simulink library "uplink_4c1r_carrier_seperation_4c"  (Simulink 8.7)
settings: Solver=ode45  StartTime=0.0  StopTime=10.0  RelTol=1e-3
undefined symbols (not defined in the file or in its folder): AdvDSPBChannelOutDisplay, dspba_ChannelInVis, dspba_ChannelOutVis, dspba_internal_get_channel_ports, dspba_internal_get_demux_ports, latency, value
libraries: DSPBAPrim x11, IQ_Square x4
settings Model: Creator=bigcat  LastModifiedBy=5g

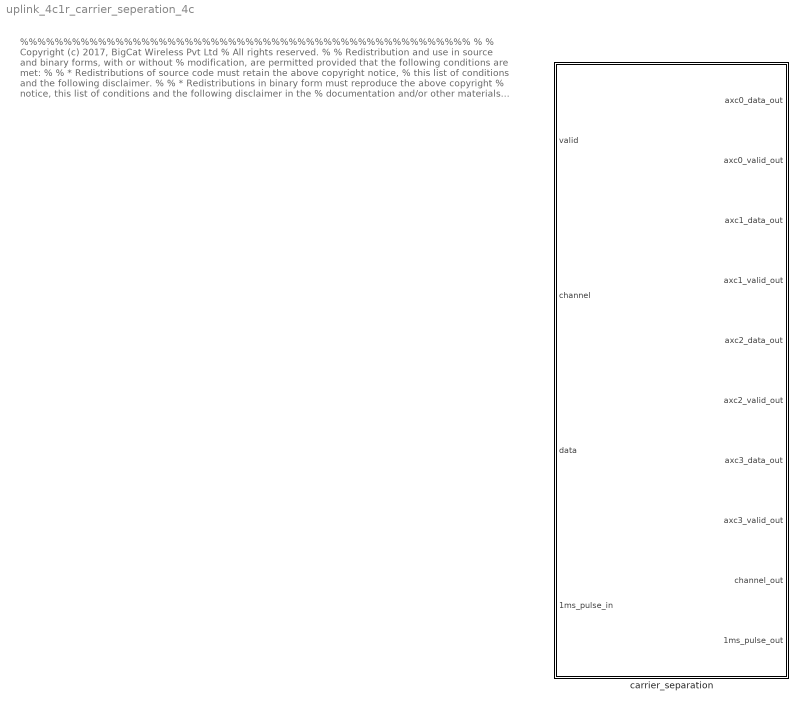
== system uplink_4c1r_carrier_seperation_4c ==
  note: %%%%%%%%%%%%%%%%%%%%%%%%%%%%%%%%%%%%%%%%%%%%%%%%%%%%
      |  %
      |  % Copyright (c) 2017, BigCat Wireless Pvt Ltd
      |  % All rights reserved.
      |  %
      |  % Redistribution and use in source and binary forms, with or without
      |  % modification, are permitted provided that the following conditions are met:
      |  %
      |  %     * Redistributions of source code must retain the above copyright notice,
      |  %       this list of conditions and the following disclaimer.
      |  %
      |  %     * Redistributions in binary form must reproduce the above copyright
      |  %       notice, this list of conditions and the following disclaimer in the
      |  %       documentation and/or other materials provided with the distribution.
      |  %
      |  %     * Neither the name of the copyright holder nor the names of its contributors
      |  %       may be used to endorse or promote products derived from this software
      |  %       without specific prior written permission.
      |  %
      |  %
      |  %
      |  % THIS SOFTWARE IS PROVIDED BY THE COPYRIGHT HOLDERS AND CONTRIBUTORS "AS IS"
      |  % AND ANY EXPRESS OR IMPLIED WARRANTIES, INCLUDING, BUT NOT LIMITED TO, THE
      |  % IMPLIED WARRANTIES OF MERCHANTABILITY AND FITNESS FOR A PARTICULAR PURPOSE ARE
      |  % DISCLAIMED. IN NO EVENT SHALL THE COPYRIGHT HOLDER OR CONTRIBUTORS BE LIABLE
      |  % FOR ANY DIRECT, INDIRECT, INCIDENTAL, SPECIAL, EXEMPLARY, OR CONSEQUENTIAL
      |  % DAMAGES (INCLUDING, BUT NOT LIMITED TO, PROCUREMENT OF SUBSTITUTE GOODS OR
      |  % SERVICES; LOSS OF USE, DATA, OR PROFITS; OR BUSINESS INTERRUPTION) HOWEVER
      |  % CAUSED AND ON ANY THEORY OF LIABILITY, WHETHER IN CONTRACT, STRICT LIABILITY,
      |  % OR TORT (INCLUDING NEGLIGENCE OR OTHERWISE) ARISING IN ANY WAY OUT OF THE USE
      |  % OF THIS SOFTWARE, EVEN IF ADVISED OF THE POSSIBILITY OF SUCH DAMAGE.
      |  %
      |   %%%%%%%%%%%%%%%%%%%%%%%%%%%%%%%%%%%%%%%%%%%%%%%%%%%%%
  carrier_separation : Subsystem  mask{Latency=0}
      mask Display:
      | disp('CARRIER_SEPERATION');
      | port_label('input',1,'v');
      | port_label('input',2,'c');
      | port_label('input',3,'d');
      | port_label('input',4,'pulse_in');
      | port_label('output',1,'q_carr1');
      | port_label('output',2,'qv_carr1');
      | port_label('output',3,'q_carr2');
      | port_label('output',4,'qv_carr2');
      | port_label('output',5,'q_carr3');
      | port_label('output',6,'qv_carr3');
      | port_label('output',7,'q_carr4');
      | port_label('output',8,'qv_carr4');
      | port_label('output',9,'qc');
      | port_label('output',10,'q_pulse');

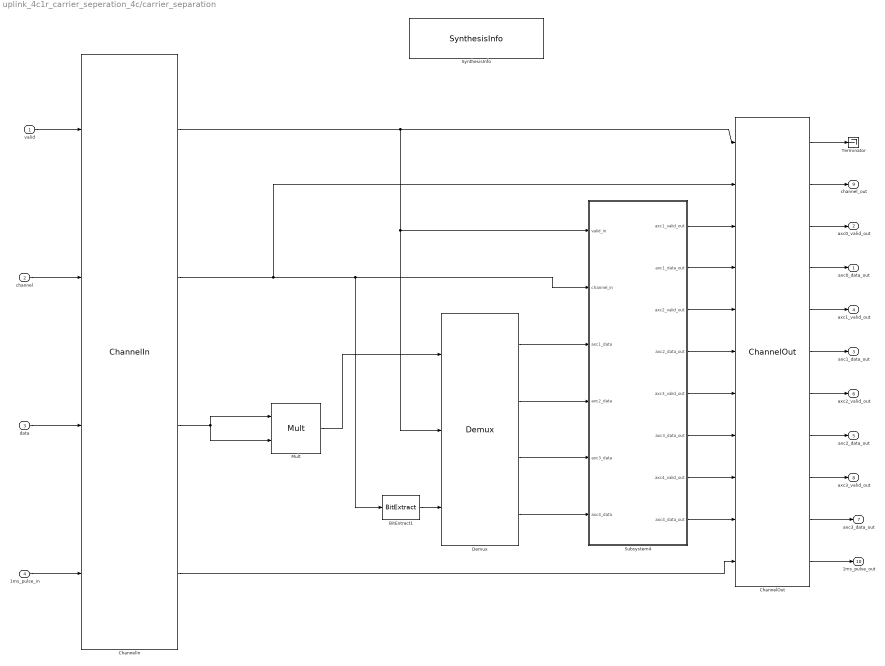
== system uplink_4c1r_carrier_seperation_4c/carrier_separation ==
  valid : Inport
  channel : Inport  Port=2
  "data " : Inport  Port=3
  "1ms_pulse_in " : Inport  Port=4
  BitExtract1 : DSPBAPrim/BitExtract  primtype=bitextract  nInputs=1  nOutputs=1  omode=Specify via dialog  otype=ufix(4)  scale=2^0  rndmethod=Unbiased  factor=1  satmethod=Symmetric  shift_vec=[0 1 2 -1]  value=1  inPortNames=[' '; ' ';]  outPortNames=[' ']  dspbaimage=dspba_prim.jpg  text=fprintf('..%d', value);  style=Optimised  visibilities=8 + 1024  version=20090407
  ChannelIn : DSPBAPrim/ChannelIn  primtype=channelin  nInputs=dspba_internal_get_channel_ports(gcb)  nOutputs=dspba_internal_get_channel_ports(gcb)  omode=Inherit via internal rule  otype=sfix(16)  scale=2^-15  rndmethod=Unbiased  factor=1  satmethod=Symmetric  shift_vec=[0 1 2 -1]  value=2  inPortNames=['v'; 'c'; '0'; '1'; '2'; '3'; '4'; '5'; '6'; '7'; '8'; '9'; 'A'; 'B'; 'D'; 'E'; 'F'; 'G'; 'H'; 'I'; 'J'; 'K'; 'L'; 'M'; 'N'; 'O'; 'P'; 'Q'; 'R'; 'S'; 'T'; 'U'; 'W'; 'X'; 'Y'; 'Z']  outPortNames=['v'; 'c'; '0'; '1'; '2'; '3'; '4'; '5'; '6'; '7'; '8'; '9'; 'A'; 'B'; 'D'; 'E'; 'F'; 'G'; 'H'; 'I'; 'J'; 'K'; 'L'; 'M'; 'N'; 'O'; 'P'; 'Q'; 'R'; 'S'; 'T'; 'U'; 'W'; 'X'; 'Y'; 'Z']  dspbaimage=dspba_prim.jpg  text=fprintf('In');  style=Optimised  dataSignals=2  foldingEnabled=off  channels=1  sampleRate=200  packetBeginPresent=off  packetBeginEnabled=off  visibilities=dspba_ChannelInVis(gcb)  latencyCorrection=0  version=20141013
  ChannelOut : DSPBAPrim/ChannelOut  primtype=channelout  nInputs=dspba_internal_get_channel_ports(gcb)  nOutputs=dspba_internal_get_channel_ports(gcb)  omode=Inherit via internal rule  otype=sfix(16)  scale=2^-15  rndmethod=Unbiased  factor=1  satmethod=Symmetric  shift_vec=[0 1 2 -1]  value=9  inPortNames=['v'; 'c'; '0'; '1'; '2'; '3'; '4'; '5'; '6'; '7'; '8'; '9'; 'A'; 'B'; 'D'; 'E'; 'F'; 'G'; 'H'; 'I'; 'J'; 'K'; 'L'; 'M'; 'N'; 'O'; 'P'; 'Q'; 'R'; 'S'; 'T'; 'U'; 'W'; 'X'; 'Y'; 'Z']  outPortNames=['v'; 'c'; '0'; '1'; '2'; '3'; '4'; '5'; '6'; '7'; '8'; '9'; 'A'; 'B'; 'D'; 'E'; 'F'; 'G'; 'H'; 'I'; 'J'; 'K'; 'L'; 'M'; 'N'; 'O'; 'P'; 'Q'; 'R'; 'S'; 'T'; 'U'; 'W'; 'X'; 'Y'; 'Z']  dspbaimage=dspba_prim.jpg  text=fprintf('Out%s', AdvDSPBChannelOutDisplay(latency));  style=Optimised  dataSignals=9  foldingEnabled=off  channels=1  sampleRate=200  packetBeginPresent=off  packetBeginEnabled=off  visibilities=dspba_ChannelOutVis(gcb)  latency=21  latencyCorrection=0  version=20141013
  Demux : DSPBAPrim/Demux  primtype=demux  nInputs=3  nOutputs=dspba_internal_get_demux_ports(gcb)  omode=Inherit via internal rule  otype=sfix(16)  scale=2^-15  rndmethod=Unbiased  factor=1  satmethod=Symmetric  shift_vec=[0 1 2 3]  value=4  inPortNames=['q'; 'v'; 'c']  outPortNames=['c0'; 'c1']  dspbaimage=dspba_prim.jpg  text=fprintf('demux');  style=Optimised  visibilities=1536  version=20100120
  Mult : DSPBAPrim/Mult  primtype=mult  nInputs=2  nOutputs=1  omode=Inherit via internal rule  otype=sfix(16)  scale=2^-15  rndmethod=Unbiased  factor=1  satmethod=Symmetric  shift_vec=[0 1 2 -1]  value=0  inPortNames=[' '; ' ';]  outPortNames=[' ']  dspbaimage=dspba_prim.jpg  text=fprintf('X');  style=Optimised  visibilities=8+2^18+2^19  floatPrecision=float32_m23  floatRounding=correct  advOptions=[]  version=20130115
  Subsystem4 : Subsystem
  SynthesisInfo : DSPBAPrim/SynthesisInfo  primtype=synthinfo  nInputs=0  nOutputs=0  omode=Inherit via internal rule  otype=sfix(16)  scale=2^-15  rndmethod=Truncate  factor=1  satmethod=Symmetric  shift_vec=[0 1 2 -1]  value=99  inPortNames=[' '; ' ';]  outPortNames=[' ']  dspbaimage=dspba_prim_ctrl.jpg  text=fprintf('Style=%s', style);  style=Scheduled  visibilities=32768  constraintInUse=on  constraintRelation=>  constraintLimit=Latency  bitAccurate=off  version=20090407
  Terminator : Terminator
  "axc0_data_out " : Outport
  axc0_valid_out : Outport  Port=2
  axc1_data_out : Outport  Port=3
  axc1_valid_out : Outport  Port=4
  axc2_data_out : Outport  Port=5
  axc2_valid_out : Outport  Port=6
  axc3_data_out : Outport  Port=7
  axc3_valid_out : Outport  Port=8
  channel_out : Outport  Port=9
  1ms_pulse_out : Outport  Port=10
  wires:
  "1ms_pulse_in "/1 -> ChannelIn/4
  ChannelOut/11 -> 1ms_pulse_out/1
  ChannelIn/4 -> ChannelOut/11
  ChannelOut/10 -> axc3_data_out/1
  ChannelOut/8 -> axc2_data_out/1
  ChannelOut/7 -> axc2_valid_out/1
  ChannelOut/6 -> axc1_data_out/1
  ChannelOut/5 -> axc1_valid_out/1
  ChannelOut/3 -> axc0_valid_out/1
  ChannelOut/9 -> axc3_valid_out/1
  ChannelOut/4 -> "axc0_data_out "/1
  ChannelIn/2 -> Subsystem4/2(channel_in), BitExtract1/1, ChannelOut/2
  ChannelIn/1 -> Demux/2, Subsystem4/1(valid_in), ChannelOut/1
  Mult/1 -> Demux/1
  BitExtract1/1 -> Demux/3
  channel/1 -> ChannelIn/2
  valid/1 -> ChannelIn/1
  ChannelOut/1 -> Terminator/1
  "data "/1 -> ChannelIn/3
  ChannelOut/2 -> channel_out/1
  ChannelIn/3 -> Mult/1, Mult/2
  Demux/1 -> Subsystem4/3(axc1_data)
  Demux/2 -> Subsystem4/4(axc2_data)
  Demux/3 -> Subsystem4/5(axc3_data)
  Demux/4 -> Subsystem4/6(axc4_data)
  Subsystem4/1(axc1_valid_out) -> ChannelOut/3
  Subsystem4/2("axc1_data_out ") -> ChannelOut/4
  Subsystem4/3(axc2_valid_out) -> ChannelOut/5
  Subsystem4/4(axc2_data_out) -> ChannelOut/6
  Subsystem4/5(axc3_valid_out) -> ChannelOut/7
  Subsystem4/6(axc3_data_out) -> ChannelOut/8
  Subsystem4/7(axc4_valid_out) -> ChannelOut/9
  Subsystem4/8(axc4_data_out) -> ChannelOut/10

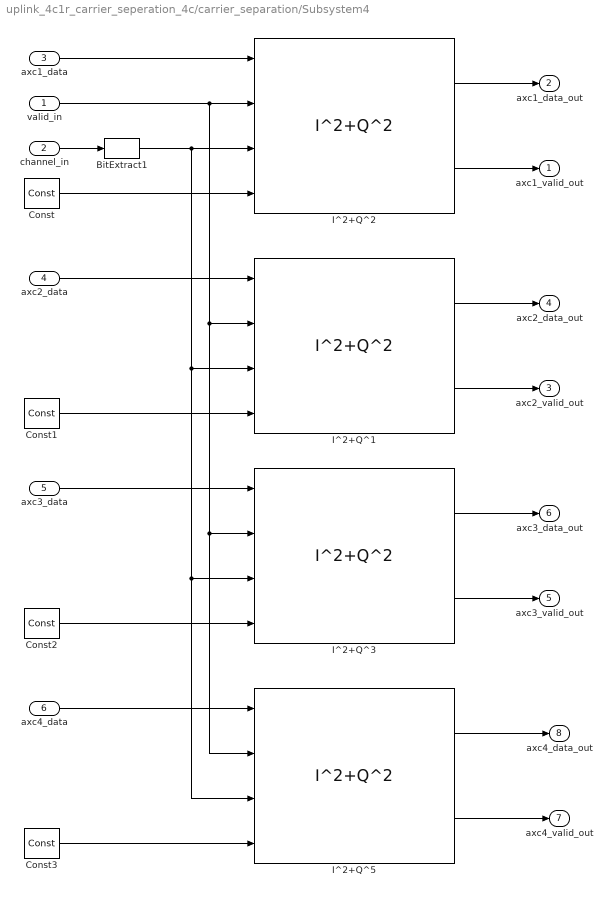
== system uplink_4c1r_carrier_seperation_4c/carrier_separation/Subsystem4 ==
  valid_in : Inport
  channel_in : Inport  Port=2
  axc1_data : Inport  Port=3
  axc2_data : Inport  Port=4
  axc3_data : Inport  Port=5
  axc4_data : Inport  Port=6
  BitExtract1 : DSPBAPrim/BitExtract  primtype=bitextract  nInputs=1  nOutputs=1  omode=Specify via dialog  otype=ufix(4)  scale=2^0  rndmethod=Unbiased  factor=1  satmethod=Symmetric  shift_vec=[0 1 2 -1]  value=1  inPortNames=[' '; ' ';]  outPortNames=[' ']  dspbaimage=dspba_prim.jpg  text=fprintf('..%d', value);  style=Optimised  visibilities=8 + 1024  version=20090407
  Const : DSPBAPrim/Const  primtype=const  nInputs=0  nOutputs=1  omode=Inherit via internal rule  otype=sfix(16)  scale=2^-15  rndmethod=Unbiased  factor=1  satmethod=Symmetric  shift_vec=[0 1 2 -1]  value=0  inPortNames=['+'; '+';]  outPortNames=[' ']  dspbaimage=dspba_prim.jpg  text=fprintf('%s', num2str(value));  style=Optimised  visibilities=8 + 1024  floatPrecision=float32_m23  version=20120820
  Const1 : DSPBAPrim/Const  primtype=const  nInputs=0  nOutputs=1  omode=Inherit via internal rule  otype=sfix(16)  scale=2^-15  rndmethod=Unbiased  factor=1  satmethod=Symmetric  shift_vec=[0 1 2 -1]  value=1  inPortNames=['+'; '+';]  outPortNames=[' ']  dspbaimage=dspba_prim.jpg  text=fprintf('%s', num2str(value));  style=Optimised  visibilities=8 + 1024  floatPrecision=float32_m23  version=20120820
  Const2 : DSPBAPrim/Const  primtype=const  nInputs=0  nOutputs=1  omode=Inherit via internal rule  otype=sfix(16)  scale=2^-15  rndmethod=Unbiased  factor=1  satmethod=Symmetric  shift_vec=[0 1 2 -1]  value=2  inPortNames=['+'; '+';]  outPortNames=[' ']  dspbaimage=dspba_prim.jpg  text=fprintf('%s', num2str(value));  style=Optimised  visibilities=8 + 1024  floatPrecision=float32_m23  version=20120820
  Const3 : DSPBAPrim/Const  primtype=const  nInputs=0  nOutputs=1  omode=Inherit via internal rule  otype=sfix(16)  scale=2^-15  rndmethod=Unbiased  factor=1  satmethod=Symmetric  shift_vec=[0 1 2 -1]  value=3  inPortNames=['+'; '+';]  outPortNames=[' ']  dspbaimage=dspba_prim.jpg  text=fprintf('%s', num2str(value));  style=Optimised  visibilities=8 + 1024  floatPrecision=float32_m23  version=20120820
  I^2+Q^{1..3,5} (4 alike) : IQ_Square/I^2+Q^2  clk=0
  axc1_valid_out : Outport
  "axc1_data_out " : Outport  Port=2
  axc2_valid_out : Outport  Port=3
  axc2_data_out : Outport  Port=4
  axc3_valid_out : Outport  Port=5
  axc3_data_out : Outport  Port=6
  axc4_valid_out : Outport  Port=7
  axc4_data_out : Outport  Port=8
  wires:
  I^2+Q^5/1 -> axc4_data_out/1
  I^2+Q^3/1 -> axc3_data_out/1
  I^2+Q^1/1 -> axc2_data_out/1
  I^2+Q^1/2 -> axc2_valid_out/1
  I^2+Q^3/2 -> axc3_valid_out/1
  channel_in/1 -> BitExtract1/1
  valid_in/1 -> I^2+Q^3/2, I^2+Q^5/2, I^2+Q^1/2, I^2+Q^2/2
  Const/1 -> I^2+Q^2/4
  axc1_data/1 -> I^2+Q^2/1
  Const1/1 -> I^2+Q^1/4
  axc2_data/1 -> I^2+Q^1/1
  BitExtract1/1 -> I^2+Q^3/3, I^2+Q^5/3, I^2+Q^1/3, I^2+Q^2/3
  Const2/1 -> I^2+Q^3/4
  Const3/1 -> I^2+Q^5/4
  I^2+Q^2/1 -> "axc1_data_out "/1
  I^2+Q^2/2 -> axc1_valid_out/1
  I^2+Q^5/2 -> axc4_valid_out/1
  axc3_data/1 -> I^2+Q^3/1
  axc4_data/1 -> I^2+Q^5/1
